simulink model "digital_filter_100Hz"  (Simulink 6.2)
settings: Solver=ode45  StartTime=0.0  StopTime=1  RelTol=1e-3
libraries: dspsigops x4, dsparch4 x1, dspsrcs4 x1
settings Model: LastModifiedBy=PHYSICS
settings DebuggingCC: SolverPrmCheckMsg=warning

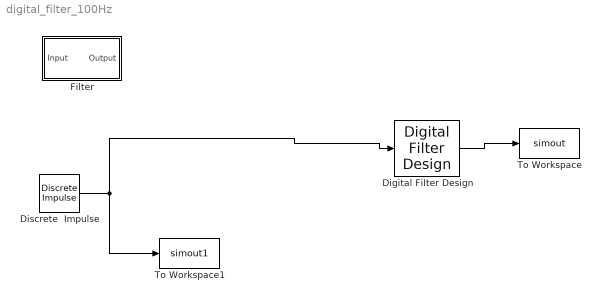
== system digital_filter_100Hz ==
  Digital Filter Design : dsparch4/Digital Filter Design  mwdsp_browser_bugfix_var=off
  Discrete  Impulse : dspsrcs4/Discrete  Impulse  Delay=0  SampleTime=1/20000  FrameSample=1  dataType=double  isSigned=on  wordLen=16  udDataType=sfix(16)  fracBitsMode=Best precision  numFracBits=15
  Filter : Subsystem  Tag=FilterWizardSubSystem
      settings: ErrorFcn=dspFilterRealizedInBasicElemsAlgLoopErrFcnCallback
  To Workspace : ToWorkspace  VariableName=simout  SampleTime=-1  SaveFormat=Array
  To Workspace1 : ToWorkspace  VariableName=simout1  SampleTime=-1  SaveFormat=Array
  wires:
  Digital Filter Design/1 -> To Workspace/1
  Discrete  Impulse/1 -> Digital Filter Design/1, To Workspace1/1

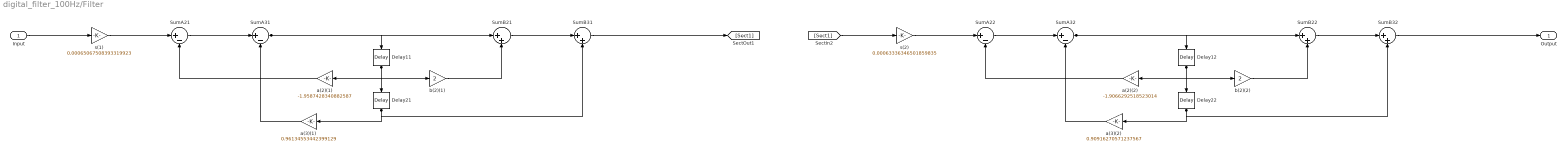
== system digital_filter_100Hz/Filter ==
  Input : Inport  Port=1  LatchInput=off
  Delay{11..12,21..22} (4 alike) : dspsigops/Delay  Orientation=down  dly_unit=Samples  delay=1  ic_detail=off  dif_ic_for_ch=off  dif_ic_for_dly=off  ic=0  reset_popup=None
  SumA{21..22,31..32} (4 alike) : Sum  Inputs=|+-  SaturateOnIntegerOverflow=on  InputSameDT=on
  SumB{21..22,31..32} (4 alike) : Sum  Inputs=|++  SaturateOnIntegerOverflow=on  InputSameDT=on
  a(2)(1) : Gain  Orientation=left  Gain=-1.9587428340882587  SaturateOnIntegerOverflow=on
  a(2)(2) : Gain  Orientation=left  Gain=-1.9066292518523014  SaturateOnIntegerOverflow=on
  a(3)(1) : Gain  Orientation=left  Gain=0.96134553442399129  SaturateOnIntegerOverflow=on
  a(3)(2) : Gain  Orientation=left  Gain=0.90916270571237567  SaturateOnIntegerOverflow=on
  b(2)(1) : Gain  Gain=2  SaturateOnIntegerOverflow=on
  b(2)(2) : Gain  Gain=2  SaturateOnIntegerOverflow=on
  s(1) : Gain  Gain=0.00065067508393319923  SaturateOnIntegerOverflow=on
  s(2) : Gain  Gain=0.00063336346501859835  SaturateOnIntegerOverflow=on
  Output : Outport
  wires:
  Input/1 -> s(1)/1
  s(1)/1 -> SumA21/1
  SumA21/1 -> SumA31/1
  SumA31/1 -> SumB21/1, Delay11/1
  SumB21/1 -> SumB31/1
  SumB31/1 -> [Sect1]
  a(2)(1)/1 -> SumA21/2
  Delay11/1 -> a(2)(1)/1, b(2)(1)/1, Delay21/1
  b(2)(1)/1 -> SumB21/2
  a(3)(1)/1 -> SumA31/2
  Delay21/1 -> a(3)(1)/1, SumB31/2
  [Sect1] -> s(2)/1
  s(2)/1 -> SumA22/1
  SumA22/1 -> SumA32/1
  SumA32/1 -> SumB22/1, Delay12/1
  SumB22/1 -> SumB32/1
  SumB32/1 -> Output/1
  a(2)(2)/1 -> SumA22/2
  Delay12/1 -> a(2)(2)/1, b(2)(2)/1, Delay22/1
  b(2)(2)/1 -> SumB22/2
  a(3)(2)/1 -> SumA32/2
  Delay22/1 -> a(3)(2)/1, SumB32/2
